simulink model "Project_sinePWM_with_PI_controller_19b"  (R2019b)
settings: Solver=ode4  StartTime=0  StopTime=1  FixedStep=5e-6  MaxStep=1e-6  RelTol=1e-6  AbsTol=1e-6  EnableMultiTasking=on
PreLoadFcn:
  | assignin('base','Ts',[5e-6])
values from neighbouring files (symbols this model uses):
  integral_term = .025    (= 0.025)    [PI_contolled_pwm_part3.m]    (also in PI_controlled_pwm.m; PI_controlled_sinpwm.m; motor3.m = 1)
  proportional_term = 10    [PI_contolled_pwm_part3.m]    (also in PI_controlled_pwm.m; PI_controlled_sinpwm.m = 50; motor3.m = 1)
undefined symbols (not defined in the file or in its folder): powergui
libraries: powerlib x13, powerlib_meascontrol x3
Description:
  | This example illustrates use of the BLDC in a closed-loop
  | speed and voltage control on a 1 kW, 3000 rpm industrial motor
  | 
  | 
  | Copyright 2008-2017 The MathWorks, Inc.
settings Model: ExtModeAutoUpdateStatusClock=off  Creator=MathWorks  LastModifiedBy=gapaul
settings SolverCC: AutoScaleAbsTol=off
settings DataIOCC: LimitDataPoints=on  SaveFormat=Array  SignalLoggingSaveFormat=ModelDataLogs  ReturnWorkspaceOutputs=off  SignalLoggingName=sigsOut
settings OptimizationCC: ExpressionDepthLimit=2147483647  InitFltsAndDblsToZero=on  LifeSpan=inf
settings DebuggingCC: UnderspecifiedInitializationDetection=Classic  MergeDetectMultiDrivingBlocksExec=none  SignalResolutionControl=TryResolveAllWithWarning  MultiTaskDSMMsg=warning  MultiTaskCondExecSysMsg=none  FcnCallInpInsideContextMsg=warning  StateNameClashWarn=warning  SFUnexpectedBacktrackingDiag=warning  SFNoUnconditionalDefaultTransitionDiag=warning  SFExecutionAtInitializationDiag=none  ArithmeticOperatorsInVariantConditions=warning
settings HardwareCC: ProdBitPerPointer=32  ProdBitPerSizeT=32  ProdBitPerPtrDiffT=32  ProdLargestAtomicFloat=None  ProdIntDivRoundTo=Undefined  ProdEndianess=Unspecified  ProdWordSize=32  ProdHWDeviceType=32-bit Generic  TargetUnknown=on
settings ModelReferenceCC: PropagateSignalLabelsOutOfModel=off
settings SFSimCC: SimUseLocalCustomCode=off  CustomCodeUndefinedFunction=UseInterfaceOnly
settings RTWCC: RTWUseLocalCustomCode=off
settings CodeAppCC: StateflowObjectComments=on
settings GRTTargetCC: TargetLangStandard=C89/C90 (ANSI)  CombineOutputUpdateFcns=off  GRTInterface=on
settings ConfigComp: CovMetricSettings=dw  CovHtmlReporting=on  CovSaveCumulativeToWorkspaceVar=on  CovSaveSingleToWorkspaceVar=on  CovExternalEMLEnable=off  CovSFcnEnable=off
settings SimscapeCC: SimscapeNormalizeSystem=off

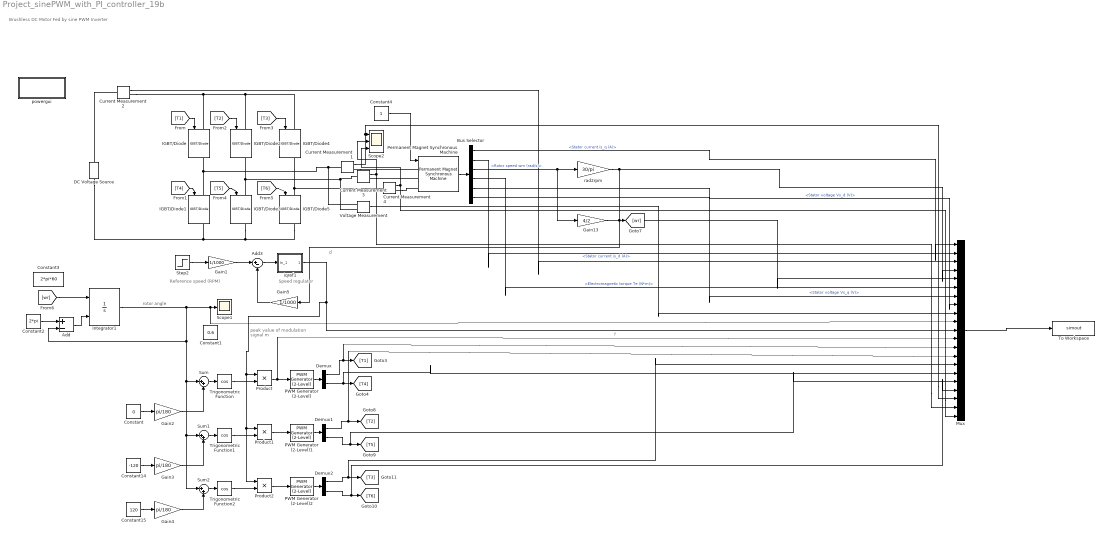
== system Project_sinePWM_with_PI_controller_19b ==
  note: peak value of modulation signal m
  note: Brushless DC Motor Fed by sine PWM Inverter
  note: rotor angle
  note: Reference
      | speed (RPM)
  note: Speed
      | regulator
  note: d
  Add : Sum  Inputs=+-
  Add3 : Sum  Inputs=|+-
  Bus Selector : BusSelector  OutputSignals=Stator current is_q (A),Stator current is_d (A),Rotor speed wm (rad/s),Electromagnetic torque Te (N*m),Stator voltage Vs_q (V),Stator voltage Vs_d (V)
  Constant : Constant  Value=0
  Constant1 : Constant  Value=0.6
  Constant14 : Constant  Value=-120
  Constant15 : Constant  Value=120
  Constant2 : Constant  Value=2*pi
  Constant3 : Constant  Value=2*pi*60
  Constant4 : Constant
  Current Measurement{1..4} (4 alike) : powerlib/Measurements/Current Measurement  PhasorSimulation=off  OutputType=Complex  PSBequivalent=0
  DC Voltage Source : powerlib/Electrical Sources/DC Voltage Source  Amplitude=72  Measurements=None
  Demux : Demux  Outputs=2
  Demux1 : Demux  Outputs=2
  Demux2 : Demux  Outputs=2
  Gain1 : Gain  Gain=1/1000
  Gain13 : Gain  Gain=4/2
  Gain2 : Gain  Gain=pi/180
  Gain3 : Gain  Gain=pi/180
  Gain4 : Gain  Gain=pi/180
  Gain5 : Gain  Gain=1/1000
  IGBT/Diode{,1..5} (6 alike) : powerlib/Power Electronics/IGBT//Diode  Ron=1e-5  Rs=1e5  Cs=inf  Measurements=on
  Integrator1 : Integrator  ExternalReset=falling
  Mux : Mux  Inputs=21
  PWM Generator (2-Level) : powerlib_meascontrol/Pulse & Signal Generators/PWM Generator (2-Level)  ModulatorType=Single-phase half-bridge (2 pulses)  ModulatorMode=Unsynchronized  Fc=1620  Pc=90  nF=30  MinMax="[ -1  1 ]"  SamplingTechnique=Natural  ModulatingSignals=off  m=0.8  Freq=60  Phase=0  Ts=5e-6  ShowCarrierOutport=off
  PWM Generator (2-Level)1 : powerlib_meascontrol/Pulse & Signal Generators/PWM Generator (2-Level)  ModulatorType=Single-phase half-bridge (2 pulses)  ModulatorMode=Unsynchronized  Fc=1620  Pc=90  nF=30  MinMax="[ -1  1 ]"  SamplingTechnique=Natural  ModulatingSignals=off  m=0.8  Freq=60  Phase=0  Ts=5e-6  ShowCarrierOutport=off
  PWM Generator (2-Level)2 : powerlib_meascontrol/Pulse & Signal Generators/PWM Generator (2-Level)  ModulatorType=Single-phase half-bridge (2 pulses)  ModulatorMode=Unsynchronized  Fc=1620  Pc=90  nF=30  MinMax="[ -1  1 ]"  SamplingTechnique=Natural  ModulatingSignals=off  m=0.8  Freq=60  Phase=0  Ts=5e-6  ShowCarrierOutport=off
  Permanent Magnet Synchronous Machine : powerlib/Machines/Permanent Magnet Synchronous Machine  NbPhases=3  FluxDistribution=Sinusoidal  RotorType=Round  MechanicalLoad=Torque Tm  PresetModel=No  ShowDetailedParameters=on  MeasurementBus=off  Resistance=3.4  Inductance=8.5e-3  dqInductances=[8.5e-3, 8.5e-3]  La=(1.1 + 3/2*11)*1e-3  MachineConstant=Flux linkage established by magnets (V.s)  Flux=0.2  VoltageCst=72.552  TorqueCst=0.6  Flat=120  Mechanical=[5e-4, 0 2]  PolePairs=4  InitialConditions=[0,0, 0,0]  InitialConditions5ph=[0 0 0 0 0 0]  RefAngle=90 degrees behind phase A axis (modified Park)  IterativeDiscreteModel=Trapezoidal non iterative  TsBlock=-1  TsPowergui=0
  Product : Product
  Product1 : Product
  Product2 : Product
  Scope1 : Scope
  Scope2 : Scope  NumInputPorts=3
  Step2 : Step  Time=0.5  Before=600  After=400  SampleTime=0
  Sum : Sum  Inputs=|++
  Sum1 : Sum  Inputs=|++
  Sum2 : Sum  Inputs=|++
  To Workspace : ToWorkspace  VariableName=simout  SaveFormat=Timeseries  SampleTime=-1
  Trigonometric Function : Trigonometry  Operator=cos
  Trigonometric Function1 : Trigonometry  Operator=cos
  Trigonometric Function2 : Trigonometry  Operator=cos
  Voltage Measurement : powerlib/Measurements/Voltage Measurement  PhasorSimulation=off  OutputType=Complex  PSBequivalent=0
  iqref1 : Subsystem  mask(PI Controller){I=integral_term, P=proportional_term, sat=[-10000, 10000]}
      mask prompts: I "Integral"; P "Proportional:"; sat "Minimum and maximum outputs:"
      mask init:
      | min=sat(1);max=sat(2);
      mask Display: disp('PI')
  powergui : Subsystem  Priority=2  AncestorBlock=powerlib/powergui  DialogController=POWERSYS.PowerSysDialog  InitFcn=powergui( 'InitFcn_Callback' , gcb , 0 , [ ] );  mask(PSB option menu block){SimulationMode=Discrete, SampleTime=5e-6, frequency=60, Iterations=50, frequencyindice=0, Pbase=100e6, ErrMax=1e-4, UnitsV=kV, UnitsW=MW, buscounter=0, FunctionMessages=off, echomessages=off, EnableUseOfTLC=off, CurrentSourceSwitches=off, DisableSnubberDevices=off, DisableRonSwitches=off, DisableVfSwitches=off, DisplayEquations=off, AutomaticDiscreteSolvers=off, SolverType=Tustin/Backward Euler (TBE), Interpol=off, ExternalGateDelay=off, methode=off, Ts=0, x0status=blocks, SPID=off, SwTol=0, HookPort=off, NonlinearTolerance=1e-4, nMaxIteration=100, ContinueOnMaxIteration=off, RestoreLinks=warning, ResistiveCurrentMeasurement=off, Frange=[0:2:500], Ylog=off, Xlog=on, ShowGrid=off, save=off, variable=ZData, structure=0, ZoomFFT=on, StartTime=0.0, cycles=1, DisplayStyle=1, fundamental=60, FreqAxis=off, MaxFrequency=1000, frequencyindicesteady=1, RmsSteady=1, display=off}
      mask prompts: SimulationMode "Simulation type:"; SampleTime "Sample time (s):"; frequency "Frequency (Hz):"; Iterations "Max iterations"; frequencyindice "Frequency (Hz)"; Pbase "Base power (VA)"; ErrMax "PQ tolerance (pu)"; UnitsV "Voltage units"; UnitsW "Power units"; buscounter "Load flow bus counter"; FunctionMessages "Disable Specialized Power Systems warnings"; echomessages "Display Specialized Power Systems compilation messages"; EnableUseOfTLC "Use TLC file when in Accelerator Simulation Mode and for code generation"; CurrentSourceSwitches "Disable ideal switching"; DisableSnubberDevices "Disable snubbers in switching devices"; DisableRonSwitches "Disable Ron resistances in switching devices"; DisableVfSwitches "Disable forward voltages in switching devices"; DisplayEquations "Display circuit differential equations"; AutomaticDiscreteSolvers "Automatically handle Discrete solver and Advanced tab solver settings of blocks"; SolverType "Discrete solver"; Interpol "Interpolate switching events"; ExternalGateDelay "Use time-stamped gate signals"; methode "Store switching topologies"; Ts "Buffer size (MBytes):"; x0status "Start simulation with initial electrical states from:"; SPID "Use ideal switching devices"; SwTol "Switch tolerance"; HookPort "Allow multiple powergui blocks"; NonlinearTolerance "Solver tolerance"; nMaxIteration "Maximum number of iterations"; ContinueOnMaxIteration "Continue Simulation if maximum number of iterations is reached"; RestoreLinks "Restore disabled links of Simscape Power Systems ST blocks:"; ResistiveCurrentMeasurement "Use non ideal current measurement blocks (1e-4Ohm internal resistance)"; Frange "Frequency Range"; Ylog "Log impedance"; Xlog "log Frequency"; ShowGrid "grid"; save "Save Data To Workspace"; variable "Variable Name"; structure "Structure Name (PSBFFTSCOPE)"; ZoomFFT "ZoomFFT (PSBFFTSCOPE)"; StartTime "Start Time (PSBFFTSCOPE)"; cycles "Cycles (PSBFFTSCOPE)"; DisplayStyle "Display style (PSBFFTSCOPE)"; fundamental "Fundamental (PSBFFTSCOPE)"; FreqAxis "Frequency Axis (PSBFFTSCOPE)"; MaxFrequency "Max Frequency (PSBFFTSCOPE)"; frequencyindicesteady "Frequency indice (STEADYSTATE)"; RmsSteady "RMS display (STEADYSTATE)"; display "Display Results"
      mask help: Set simulation type, simulation parameters, and preferences.
      mask init:
      | dispMessage = powergui('MaskInitialization',gcb,SimulationMode,SampleTime);
      settings: PreSaveFcn=powergui( 'PreSaveFcn_Callback' , gcb , [ ] , [ ] );  OpenFcn=sps_rtmsupport('OpenFcn',gcbh)
      mask Help: helpview(psbhelp)
      mask TypeOptions SimulationMode: Continuous | Discrete | Phasor | Discrete phasor
      mask Callback SimulationMode: powergui('SimulationType',[],[],gcb);
      mask TypeOptions UnitsV: V | kV
      mask TypeOptions UnitsW: W | kW | MW
      mask Callback CurrentSourceSwitches: powergui('SimulationType',[],[],gcb);
      mask Callback AutomaticDiscreteSolvers: powergui('SimulationType',[],[],gcb);
      mask TypeOptions SolverType: Tustin/Backward Euler (TBE) | Tustin | Backward Euler
      mask Callback SolverType: powergui('SimulationType',[],[],gcb);
      mask Callback Interpol: powergui('SimulationType',[],[],gcb);
      mask Callback ExternalGateDelay: powergui('SimulationType',[],[],gcb);
      mask Callback methode: powergui('SimulationType',[],[],gcb);
      mask TypeOptions x0status: blocks | steady | zero
      mask TypeOptions RestoreLinks: yes | warning | no
      mask Callback display: sps_rtmsupport('parametereditingmodes',gcbh) % Will be executed last in parameter callbacks to ensure mask enable consistency
      mask DialogControl SolverTab Prompt: Solver
      mask DialogControl AutoSolverNote Prompt: The Simulation type parameter is governed by Simulink. To access the Powergui solver settings, unselect auto (Automatic solver selection) solver in the Simulink solver options.
      mask DialogControl AnalysisTools Prompt: Tools
      mask DialogControl SteadyState Prompt: Steady-State
      mask DialogControl SteadyState Callback:
      | close_system(gcb)
      | power_steadystate(bdroot(gcb),gcb);
      mask DialogControl InitialState Prompt: Initial State
      mask DialogControl InitialState Callback:
      | close_system(gcb)
      | power_initstates(bdroot(gcb),gcb)
      mask DialogControl MachineInitialization Prompt: Machine Initialization
      mask DialogControl MachineInitialization Callback:
      | close_system(gcb)
      | power_loadflow(bdroot(gcb),gcb)
      mask DialogControl ImpedanceMeasurement Prompt: Impedance Measurement
      mask DialogControl ImpedanceMeasurement Callback:
      | close_system(gcb)
      | power_zmeter(bdroot(gcb),gcb)
      mask DialogControl FFTAnalysis Prompt: FFT Analysis
      mask DialogControl FFTAnalysis Callback:
      | close_system(gcb)
      | power_fftscope(bdroot(gcb),gcb)
      mask DialogControl LinearSystemAnalyzer Prompt: Use Linear System Analyzer
      mask DialogControl LinearSystemAnalyzer Callback:
      | close_system(gcb)
      | power_ltiview(bdroot(gcb),gcb)
      mask DialogControl HysteresisDesign Prompt: Hysteresis Design
      mask DialogControl HysteresisDesign Callback:
      | close_system(gcb)
      | power_hysteresis(bdroot(gcb),gcb)
      mask DialogControl RLCLineParameters Prompt: RLC Line Parameters
      mask DialogControl RLCLineParameters Callback:
      | close_system(gcb)
      | power_lineparam(bdroot(gcb),gcb)
      mask DialogControl GenerateReprot Prompt: Generate Report
      mask DialogControl GenerateReprot Callback:
      | close_system(gcb)
      | power_report(bdroot(gcb),gcb)
      mask DialogControl Control14 Prompt: Customize SPS blocks
      mask DialogControl Control14 Callback:
      | close_system(gcb);
      | power_customize;
      mask DialogControl LoadFlow Prompt: Load Flow
      mask DialogControl LoadFlow Callback:
      | close_system(gcb)
      | power_loadflow('-v2',bdroot(gcb))
      mask DialogControl Container14 Prompt: Load flow settings
      mask DialogControl ParameterTabVar012 Prompt: Preferences
      mask DialogControl Solver Prompt: Solver
      mask DialogControl SolverDetails Prompt: Solver details for nonlinear elements
      mask Display: color('blue'),disp(dispMessage)
  rad2rpm : Gain  Gain=30/pi
  wires:
  Constant4/1 -> Permanent Magnet Synchronous Machine/1
  Voltage Measurement/1 -> Mux/9
  Permanent Magnet Synchronous Machine/1 -> Bus Selector/1
  Bus Selector/3 -> Gain13/1, rad2rpm/1  "<Rotor speed wm (rad/s)>"
  Bus Selector/2 -> Mux/2  "<Stator current is_d (A)>"
  [T4] -> IGBT/Diode1/1
  [T5] -> IGBT/Diode3/1
  [T6] -> IGBT/Diode5/1
  [T1] -> IGBT/Diode/1
  [T2] -> IGBT/Diode2/1
  [T3] -> IGBT/Diode4/1
  Constant2/1 -> Add/1
  Add/1 -> Integrator1/2
  [wr] -> Integrator1/1
  Bus Selector/6 -> Mux/8  "<Stator voltage Vs_d (V)>"
  Constant/1 -> Gain2/1
  PWM Generator (2-Level)1/1 -> Demux1/1
  PWM Generator (2-Level)2/1 -> Demux2/1
  Sum1/1 -> Trigonometric Function1/1
  Gain3/1 -> Sum1/2
  Sum/1 -> Trigonometric Function/1
  Gain4/1 -> Sum2/2
  Constant14/1 -> Gain3/1
  Constant15/1 -> Gain4/1
  Gain2/1 -> Sum/2
  Sum2/1 -> Trigonometric Function2/1
  Product2/1 -> PWM Generator (2-Level)2/1
  Product/1 -> Mux/12, PWM Generator (2-Level)/1  "f"
  Product1/1 -> PWM Generator (2-Level)1/1
  Trigonometric Function2/1 -> Product2/2
  Trigonometric Function1/1 -> Product1/2
  Trigonometric Function/1 -> Product/2
  Demux/1 -> Mux/13, [T1]
  Demux/2 -> Mux/16, [T4]
  Demux2/2 -> Mux/18, [T6]
  Current Measurement4/1 -> Mux/21, Scope2/3
  Current Measurement2/1 -> Mux/3
  Bus Selector/5 -> Mux/7  "<Stator voltage Vs_q (V)>"
  Current Measurement1/1 -> Mux/19, Scope2/1
  Integrator1/1 -> Mux/10, Scope1/1, Add/2, Sum/1, Sum2/1, Sum1/1
  Demux1/2 -> Mux/17, [T5]
  rad2rpm/1 -> Gain5/1, Mux/4
  iqref1/1(Out_1) -> Product2/1, Product1/1, Product/1, Mux/11
  Gain13/1 -> Mux/5, [wr]
  Demux2/1 -> Mux/15, [T3]
  Current Measurement3/1 -> Mux/20, Scope2/2
  PWM Generator (2-Level)/1 -> Demux/1
  Bus Selector/1 -> Mux/1  "<Stator current is_q (A)>"
  Demux1/1 -> Mux/14, [T2]
  Bus Selector/4 -> Mux/6  "<Electromagnetic torque Te (N*m)>"
  Mux/1 -> To Workspace/1
  Step2/1 -> Gain1/1
  Gain5/1 -> Add3/2
  Add3/1 -> iqref1/1(In_1)
  Gain1/1 -> Add3/1
  connections:
  IGBT/Diode/RConn1 -- Current Measurement1/LConn1 -- Voltage Measurement/LConn1 -- IGBT/Diode1/LConn1
  IGBT/Diode2/RConn1 -- Current Measurement3/LConn1 -- Voltage Measurement/LConn2 -- IGBT/Diode3/LConn1
  IGBT/Diode4/RConn1 -- Current Measurement4/LConn1 -- IGBT/Diode5/LConn1
  IGBT/Diode1/RConn1 -- DC Voltage Source/LConn1 -- IGBT/Diode5/RConn1 -- IGBT/Diode3/RConn1
  IGBT/Diode2/LConn1 -- IGBT/Diode4/LConn1 -- IGBT/Diode/LConn1 -- Current Measurement2/RConn1
  Current Measurement2/LConn1 -- DC Voltage Source/RConn1
  Current Measurement1/RConn1 -- Permanent Magnet Synchronous Machine/LConn1
  Current Measurement3/RConn1 -- Permanent Magnet Synchronous Machine/LConn2
  Current Measurement4/RConn1 -- Permanent Magnet Synchronous Machine/LConn3

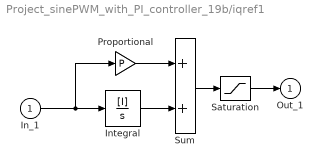
== system Project_sinePWM_with_PI_controller_19b/iqref1 ==
  In_1 : Inport
  Integral : TransferFcn  Numerator=[I]  Denominator=[1 0]
  Proportional : Gain  Gain=P  SaturateOnIntegerOverflow=on  OutDataTypeStr=Inherit: Same as input  ParamDataTypeStr=Inherit: Same as input
  Saturation : Saturate  UpperLimit=max  LowerLimit=min
  Sum : Sum  InputSameDT=on  SaturateOnIntegerOverflow=on  OutDataTypeStr=Inherit: Same as first input
  Out_1 : Outport  InitialOutput=0  VectorParamsAs1DForOutWhenUnconnected=off
  wires:
  Saturation/1 -> Out_1/1
  Sum/1 -> Saturation/1
  Proportional/1 -> Sum/1
  In_1/1 -> Proportional/1, Integral/1
  Integral/1 -> Sum/2

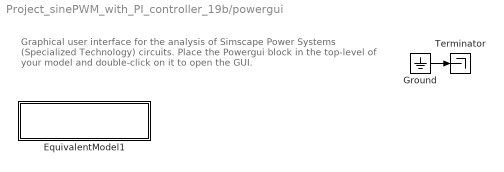
== system Project_sinePWM_with_PI_controller_19b/powergui ==
  note: Graphical user interface for the analysis of
      | Simscape Power Systems (Specialized Technology) circuits.
      | Place the Powergui block in the top-level of your model and double-click
      | on it to open the GUI.
  EquivalentModel1 : Subsystem
      mask init:
      | S  = GetDataForEquivalentModel('Discrete',gcbh);
      mask Display:
      | color('red')
      | disp('EQUIVALENT CIRCUIT\nDiscrete')
  Ground : Ground
  Terminator : Terminator
  wires:
  Ground/1 -> Terminator/1

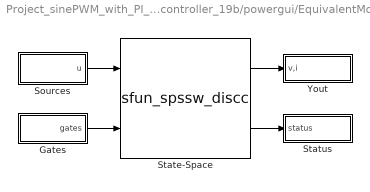
== system Project_sinePWM_with_PI_controller_19b/powergui/EquivalentModel1 ==
  Gates : Subsystem
  Sources : Subsystem
  State-Space : S-Function  FunctionName=sfun_spssw_discc  Parameters=S.Ts,S.A, S.B, S.C, S.D, S.x0, S.EnableUseOfTLC,S.SwitchResistance ,S.SwitchType, S.SwitchGateInitialValue, S.OutputsToResetToZero, S.TBEON,S.SaveMatrices,S.BufferSize  SFunctionDeploymentMode=off  EnableBusSupport=off
  Status : Subsystem
  Yout : Subsystem
  wires:
  Gates/1(gates) -> State-Space/2
  Sources/1(u) -> State-Space/1
  State-Space/2 -> Status/1(status)
  State-Space/1 -> Yout/1(v,i)

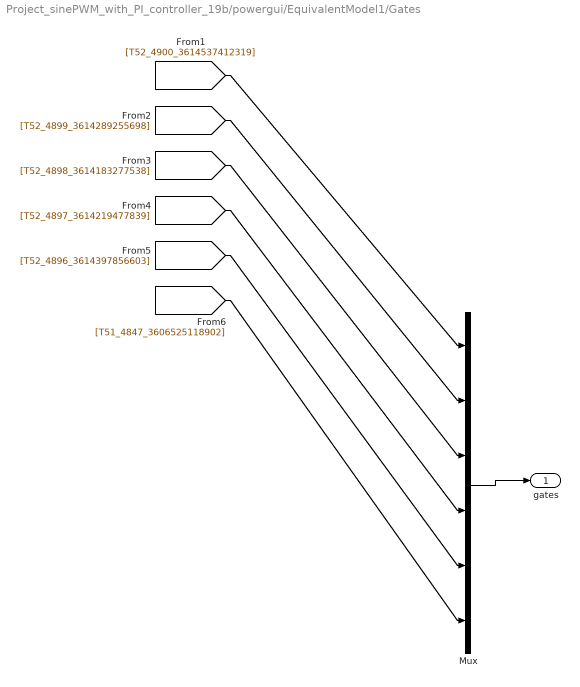
== system Project_sinePWM_with_PI_controller_19b/powergui/EquivalentModel1/Gates ==
  Mux : Mux  Inputs=[1 1 1 1 1 1]
  gates : Outport  VectorParamsAs1DForOutWhenUnconnected=off
  wires:
  Mux/1 -> gates/1
  [T52_4900_3614537412319] -> Mux/1
  [T52_4899_3614289255698] -> Mux/2
  [T52_4898_3614183277538] -> Mux/3
  [T52_4897_3614219477839] -> Mux/4
  [T52_4896_3614397856603] -> Mux/5
  [T51_4847_3606525118902] -> Mux/6

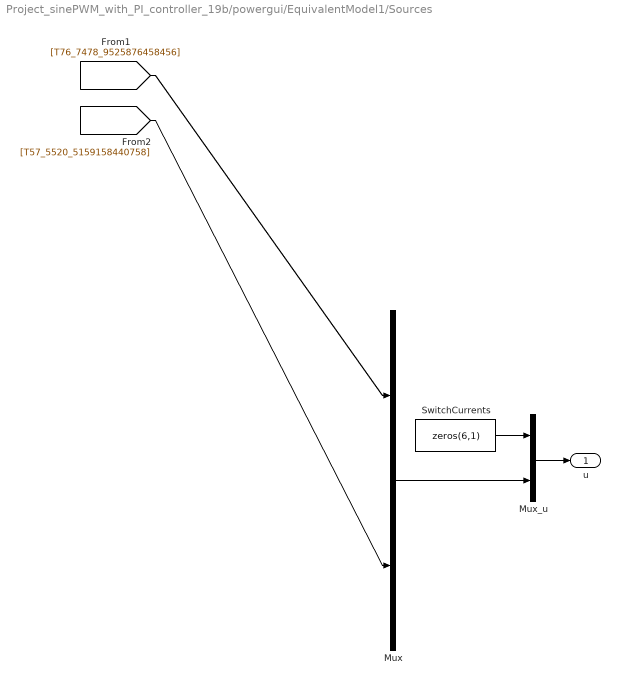
== system Project_sinePWM_with_PI_controller_19b/powergui/EquivalentModel1/Sources ==
  Mux : Mux  Inputs=[2 1]
  Mux_u : Mux  Inputs=[6 3]
  SwitchCurrents : Constant  Value=zeros(6,1)
  u : Outport  VectorParamsAs1DForOutWhenUnconnected=off
  wires:
  Mux_u/1 -> u/1
  SwitchCurrents/1 -> Mux_u/1
  Mux/1 -> Mux_u/2
  [T76_7478_9525876458456] -> Mux/1
  [T57_5520_5159158440758] -> Mux/2

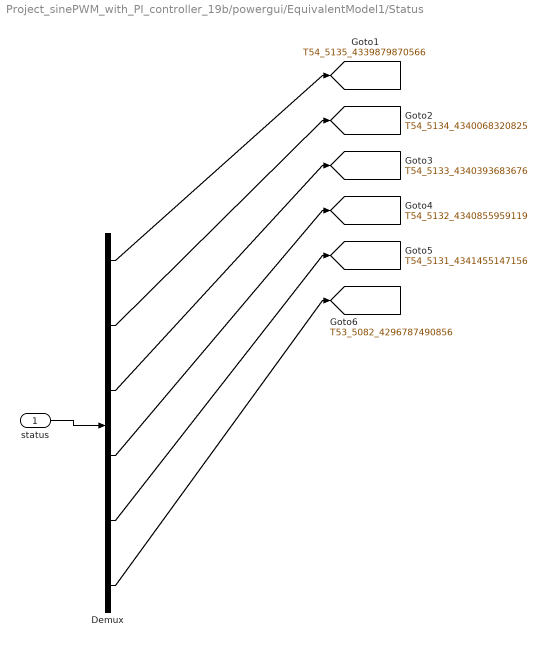
== system Project_sinePWM_with_PI_controller_19b/powergui/EquivalentModel1/Status ==
  status : Inport
  Demux : Demux  Outputs=[1 1 1 1 1 1]
  tag scope: T53_5082_4296787490856=global, T54_5131_4341455147156=global, T54_5132_4340855959119=global, T54_5133_4340393683676=global, T54_5134_4340068320825=global, T54_5135_4339879870566=global
  wires:
  status/1 -> Demux/1
  Demux/1 -> [T54_5135_4339879870566]
  Demux/2 -> [T54_5134_4340068320825]
  Demux/3 -> [T54_5133_4340393683676]
  Demux/4 -> [T54_5132_4340855959119]
  Demux/5 -> [T54_5131_4341455147156]
  Demux/6 -> [T53_5082_4296787490856]

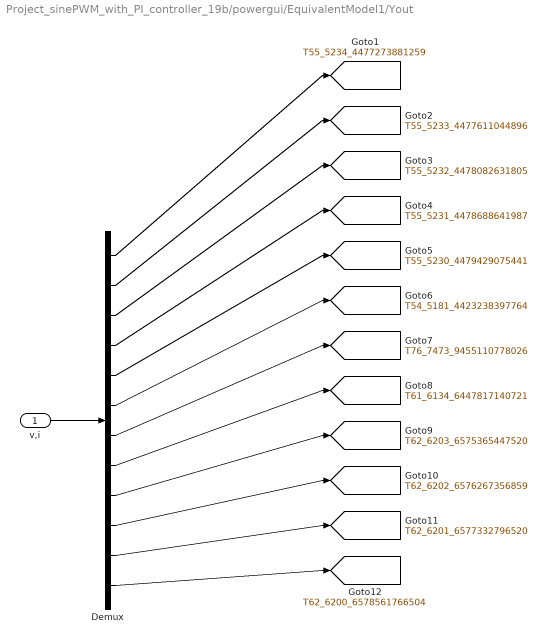
== system Project_sinePWM_with_PI_controller_19b/powergui/EquivalentModel1/Yout ==
  v,i : Inport
  Demux : Demux  Outputs=[1 1 1 1 1 1 2 1 1 1 1 1]
  tag scope: T54_5181_4423238397764=global, T55_5230_4479429075441=global, T55_5231_4478688641987=global, T55_5232_4478082631805=global, T55_5233_4477611044896=global, T55_5234_4477273881259=global, T61_6134_6447817140721=global, T62_6200_6578561766504=global, T62_6201_6577332796520=global, T62_6202_6576267356859=global, T62_6203_6575365447520=global, T76_7473_9455110778026=global
  wires:
  v,i/1 -> Demux/1
  Demux/1 -> [T55_5234_4477273881259]
  Demux/2 -> [T55_5233_4477611044896]
  Demux/3 -> [T55_5232_4478082631805]
  Demux/4 -> [T55_5231_4478688641987]
  Demux/5 -> [T55_5230_4479429075441]
  Demux/6 -> [T54_5181_4423238397764]
  Demux/7 -> [T76_7473_9455110778026]
  Demux/8 -> [T61_6134_6447817140721]
  Demux/9 -> [T62_6203_6575365447520]
  Demux/10 -> [T62_6202_6576267356859]
  Demux/11 -> [T62_6201_6577332796520]
  Demux/12 -> [T62_6200_6578561766504]
